simulink model "sampleModel254"  (R2021b)
settings: Solver=VariableStepAuto  StartTime=0.0  StopTime=10.0  RelTol=1e-3
undefined symbols (not defined in the file or in its folder): Newton, Raphson
libraries: simulink x14, slpidlib x3
settings Model: Creator=user  LastModifiedBy=user

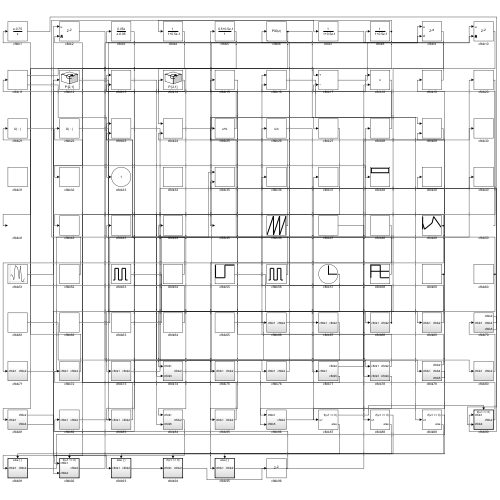
[thumbnail: Simulink's stored preview of the top-level diagram]
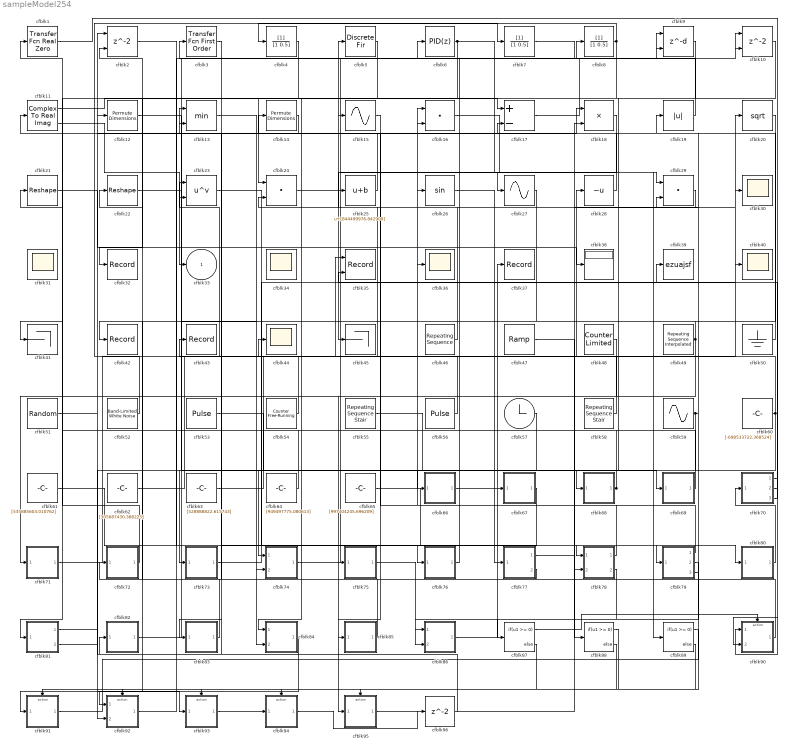
== system sampleModel254 ==
  cfblk1 : simulink/Discrete/Transfer Fcn Real Zero  ZeroZ=0.75  ICPrevInput=0.0  DoSatur=off
      settings: SourceProductBaseCode=SL
  cfblk10 : Delay  ShowEnablePort=on  SampleTime=1
      settings: InputPortMap=u0,e6
  cfblk11 : ComplexToRealImag
  cfblk12 : PermuteDimensions
  cfblk13 : MinMax  Inputs=2
  cfblk14 : PermuteDimensions
  cfblk15 : Sin  TimeSource=Use external signal  SampleTime=0
  cfblk16 : DotProduct  InputSameDT=on  OutDataTypeStr=Inherit: Inherit via internal rule
  cfblk17 : Sum  Inputs=+-
  cfblk18 : Product  Inputs=**
  cfblk19 : Abs
  cfblk2 : Delay  ShowEnablePort=on  SampleTime=1
      settings: InputPortMap=u0,e6
  cfblk20 : Sqrt  SaturateOnIntegerOverflow=on
  cfblk21 : Reshape
  cfblk22 : Reshape
  cfblk23 : Math  Operator=pow  SaturateOnIntegerOverflow=on
  cfblk24 : DotProduct  InputSameDT=on  OutDataTypeStr=Inherit: Inherit via internal rule
  cfblk25 : Bias  Bias=[844499976.842909]
  cfblk26 : Trigonometry
  cfblk27 : Sin  TimeSource=Use external signal  SampleTime=0
  cfblk28 : UnaryMinus
  cfblk29 : DotProduct  InputSameDT=on  OutDataTypeStr=Inherit: Inherit via internal rule
  cfblk3 : simulink/Discrete/Transfer Fcn First Order  PoleZ=0.95  ICPrevOutput=0.0  DoSatur=off
  cfblk{30..31,34,36,40,44} (6 alike) : Scope
      cfblk31 settings: Floating=on
      cfblk34 settings: Floating=on
  cfblk32 : Record  FileSettingsInternal="{\"entries\":[{\"content\":{\"excelSettings\":{\"content\":{},\"type\":\"Streamout.ExcelSettings\"}},\"type\":\"Streamout.FileSettingStorage\",\"uuid\":\"f8cac019-48e6-4489-905a-432bda5f2089\"}],\"packageUris\":[\"http://schema.mathworks.com/mf0/streamout_blocks/R2020a\"],\"version\":\"1.0\"}"  SignalsInternal="{\"entries\":[{\"content\":{\"signals\":[{\"content\":{\"blockPath\":[\"sampleModel254/cfblk32\"],\"channel\":[],\"dimensions\":[1],\"domain\":\"sampleModel254/cfblk32\",\"lineColor\":\"#64d413\",\"plots\":[1],\"port\":1,\"sid\":[\"\"],\"signalID\":10374,\"signalName\":\"cfblk6\"},\"type\":\"RecordBlkView.Signal\",\"uuid\":\"dce0b534-ecb6-4d5b-a233-2a280a14c64b\"}]},\"type\":\"RecordBlkView.InputSignals\",\"uuid\":\"4063d075-ef2d-4937-aee0-8c6ee8d3b7d8\"}],\"packageUris\":[\"http://schema.mathworks.com/mf0/streamout_blocks/R2020a\"],\"version\":\"1.0\"}"  VisualizationBindings="{\"sparklinesplugin\":{\"info\":[{\"bindingParametersList\":[],\"subplotID\":1}]}}"
  cfblk35 : Record  FileSettingsInternal="{\"entries\":[{\"content\":{\"excelSettings\":{\"content\":{},\"type\":\"Streamout.ExcelSettings\"}},\"type\":\"Streamout.FileSettingStorage\",\"uuid\":\"45c7964c-3e30-4dde-8807-5f474ab24dd7\"}],\"packageUris\":[\"http://schema.mathworks.com/mf0/streamout_blocks/R2020a\"],\"version\":\"1.0\"}"  Layout=[1 1]  SignalsInternal="{\"entries\":[{\"content\":{\"signals\":[{\"content\":{\"blockPath\":[\"sampleModel254/cfblk35\"],\"channel\":[],\"dimensions\":[1],\"domain\":\"sampleModel254/cfblk35\",\"lineColor\":\"#a2142f\",\"plots\":[1],\"port\":1,\"sid\":[\"\"],\"signalID\":10378,\"signalName\":\"cfblk71\"},\"type\":\"RecordBlkView.Signal\",\"uuid\":\"ef5cb758-7369-4c78-a78d-835c385c3eb8\"},{\"content\":{\"blockPath\":[\"sampleModel254/cfblk35\"],\"channel\":[],\"dimensions\":[1],\"domain\":\"sampleModel254/cfblk35\",\"lineColor\":\"#139fff\",\"plots\":[1],\"port\":2,\"sid\":[\"\"],\"signalID\":10382,\"signalName\":\"cfblk70:3\"},\"type\":\"RecordBlkView.Signal\",\"uuid\":\"7c8c1d86-132f-4531-ad7d-4a8a75f6ae5b\"}]},\"type\":\"RecordBlkView.InputSignals\",\"uuid\":\"62f64e2d-ebf5-4119-9c8a-3f565d651dbb\"}],\"packageUris\":[\"http://schema.mathworks.com/mf0/streamout_blocks/R2020a\"],\"version\":\"1.0\"}"  VisualizationBindings="{\"xyplotplugin\":{\"info\":[{\"series\":[{\"bindingParametersList\":[{\"parameter\":\"X-Axis\",\"signalID\":10378,\"signalName\":\"cfblk71\"},{\"parameter\":\"Y-Axis\",\"signalID\":10382,\"signalName\":\"cfblk70:3\"}],\"seriesID\":26922}],\"subplotID\":1}]}}"  CompatibilityTag=XY
  cfblk37 : Record  FileSettingsInternal="{\"entries\":[{\"content\":{\"excelSettings\":{\"content\":{},\"type\":\"Streamout.ExcelSettings\"}},\"type\":\"Streamout.FileSettingStorage\",\"uuid\":\"cea6e5c2-86dc-4383-be1d-b91c9e701202\"}],\"packageUris\":[\"http://schema.mathworks.com/mf0/streamout_blocks/R2020a\"],\"version\":\"1.0\"}"  SignalsInternal="{\"entries\":[{\"content\":{\"signals\":[{\"content\":{\"blockPath\":[\"sampleModel254/cfblk37\"],\"channel\":[],\"dimensions\":[1],\"domain\":\"sampleModel254/cfblk37\",\"lineColor\":\"#d95319\",\"plots\":[1],\"port\":1,\"sid\":[\"\"],\"signalID\":10394,\"signalName\":\"cfblk66\"},\"type\":\"RecordBlkView.Signal\",\"uuid\":\"769467fa-09e5-418b-a735-847f3fde8334\"}]},\"type\":\"RecordBlkView.InputSignals\",\"uuid\":\"660e46a3-809b-43d8-8dce-437cd846730a\"}],\"packageUris\":[\"http://schema.mathworks.com/mf0/streamout_blocks/R2020a\"],\"version\":\"1.0\"}"  VisualizationBindings="{\"sparklinesplugin\":{\"info\":[{\"bindingParametersList\":[],\"subplotID\":1}]}}"
  cfblk38 : Display
  cfblk39 : ToWorkspace  VariableName=ezuajsf  SaveFormat=Timeseries  SampleTime=-1
  cfblk4 : DiscreteFilter  SampleTime=1
  cfblk41 : Terminator
  cfblk42 : Record  FileSettingsInternal="{\"entries\":[{\"content\":{\"excelSettings\":{\"content\":{},\"type\":\"Streamout.ExcelSettings\"}},\"type\":\"Streamout.FileSettingStorage\",\"uuid\":\"c36e397d-8249-40e7-b36d-c436f8041f2b\"}],\"packageUris\":[\"http://schema.mathworks.com/mf0/streamout_blocks/R2020a\"],\"version\":\"1.0\"}"  SignalsInternal="{\"entries\":[{\"content\":{\"signals\":[{\"content\":{\"blockPath\":[\"sampleModel254/cfblk42\"],\"channel\":[],\"dimensions\":[1],\"domain\":\"sampleModel254/cfblk42\",\"lineColor\":\"#22b573\",\"plots\":[1],\"port\":1,\"sid\":[\"\"],\"signalID\":10386,\"signalName\":\"cfblk49\"},\"type\":\"RecordBlkView.Signal\",\"uuid\":\"95bb58e3-29ab-4543-933f-3fe3cf8075e7\"}]},\"type\":\"RecordBlkView.InputSignals\",\"uuid\":\"3d27722b-4af2-4bd2-8e99-f87c6225f507\"}],\"packageUris\":[\"http://schema.mathworks.com/mf0/streamout_blocks/R2020a\"],\"version\":\"1.0\"}"  VisualizationBindings="{\"sparklinesplugin\":{\"info\":[{\"bindingParametersList\":[],\"subplotID\":1}]}}"
  cfblk43 : Record  FileSettingsInternal="{\"entries\":[{\"content\":{\"excelSettings\":{\"content\":{},\"type\":\"Streamout.ExcelSettings\"}},\"type\":\"Streamout.FileSettingStorage\",\"uuid\":\"d18e721d-55df-43b9-9b5f-e2e7fb6a57d4\"}],\"packageUris\":[\"http://schema.mathworks.com/mf0/streamout_blocks/R2020a\"],\"version\":\"1.0\"}"  SignalsInternal="{\"entries\":[{\"content\":{\"signals\":[{\"content\":{\"blockPath\":[\"sampleModel254/cfblk43\"],\"channel\":[],\"dimensions\":[1,1],\"domain\":\"sampleModel254/cfblk43\",\"lineColor\":\"#0072bd\",\"plots\":[1],\"port\":1,\"sid\":[\"\"],\"signalID\":10390,\"signalName\":\"cfblk90\"},\"type\":\"RecordBlkView.Signal\",\"uuid\":\"5a0785be-ac31-40ab-801e-d0ec680084d0\"}]},\"type\":\"RecordBlkView.InputSignals\",\"uuid\":\"405e9301-8fb1-412e-9e94-656a63dfe870\"}],\"packageUris\":[\"http://schema.mathworks.com/mf0/streamout_blocks/R2020a\"],\"version\":\"1.0\"}"  VisualizationBindings="{\"sparklinesplugin\":{\"info\":[{\"bindingParametersList\":[],\"subplotID\":1}]}}"
  cfblk45 : Terminator
  cfblk46 : simulink/Sources/Repeating Sequence  rep_seq_t=[0 2]  rep_seq_y=[-139154258.998502, 203170849.234022]
  cfblk47 : simulink/Sources/Ramp  slope=[-2828.805781]  start=[47.728047]  InitialOutput=[-572084.834406]
  cfblk48 : simulink/Sources/Counter Limited  uplimit=[923.000000]  tsamp=-1
  cfblk49 : simulink/Sources/Repeating Sequence Interpolated  OutValues=[534969877.028503, 207347535.220771, 565089193.640656, 960177596.620139, 325028522.686949]  TimeValues=[0 0.1 0.5 0.6 1].'  LookUpMeth=Use Input Above  tsamp=0.01  OutMin=[]  OutMax=[]  OutDataTypeStr=double  OutputDataTypeScalingMode=double  OutDataType=fixdt(0,8)  OutScaling=2^-10
  cfblk5 : DiscreteFir  SampleTime=1
  cfblk50 : Ground
  cfblk51 : RandomNumber  Mean=[-71879.908599]  Variance=[65031.092299]  Seed=[190273375.000000]  SampleTime=0.1
  cfblk52 : simulink/Sources/Band-Limited White Noise  Cov=[5298985732.957167]  Ts=0.1  seed=[2012635367.000000]
  cfblk53 : DiscretePulseGenerator  PulseType=Time based  Amplitude=[128987479.442935]  Period=[95035691.423141]  PulseWidth=5  PhaseDelay=[6.000000]
  cfblk54 : simulink/Sources/Counter Free-Running  NumBits=[55.000000]  tsamp=-1
  cfblk55 : simulink/Sources/Repeating Sequence Stair  OutValues=[162166375.271766, 424616058.616663]  tsamp=-1  OutMin=[]  OutMax=[]  OutDataTypeStr=double  OutputDataTypeScalingMode=double  OutDataType=fixdt(0,8)  ConRadixGroup=Best Precision: Vector-wise  OutScaling=2^-12
  cfblk56 : DiscretePulseGenerator  PulseType=Time based  Amplitude=[530617936.673465]  Period=[21583410.222878]  PulseWidth=5  PhaseDelay=[1.000000]
  cfblk57 : Clock
  cfblk58 : simulink/Sources/Repeating Sequence Stair  OutValues=[403041999.345838, -421039062.642229]  tsamp=-1  OutMin=[]  OutMax=[]  OutDataTypeStr=double  OutputDataTypeScalingMode=double  OutDataType=fixdt(0,8)  ConRadixGroup=Best Precision: Vector-wise  OutScaling=2^-12
  cfblk59 : Sin  Amplitude=[160730542.928432]  Bias=[-895763659.447249]  SampleTime=0
  cfblk6 : slpidlib/PID Controller  Controller=PID  Form=Parallel  TimeDomain=Discrete-time  UseExternalTs=off  SampleTime=1  IntegratorMethod=Forward Euler  FilterMethod=Forward Euler  ControllerParametersSource=internal  P=1  I=1  D=0  UseFilter=on  N=100  TunerSelectOption=Transfer Function Based (PID Tuner App)  InitialConditionSource=internal  InitialConditionForIntegrator=0  InitialConditionForFilter=0  DifferentiatorICPrevScaledInput=0  ExternalReset=none  TrackingMode=off  Kt=1  LimitOutput=off  SatLimitsSource=internal  UpperSaturationLimit=inf  LowerSaturationLimit=-inf  LinearizeAsGain=off  AntiWindupMode=none  Kb=1  POutMin=[]  POutMax=[]  IOutMin=[]  IOutMax=[]  DOutMin=[]  DOutMax=[]  NOutMin=[]  NOutMax=[]  SumOutMin=[]  SumOutMax=[]  SaturationOutMin=[]  SaturationOutMax=[]  PParamMin=[]  PParamMax=[]  IParamMin=[]  IParamMax=[]  DParamMin=[]  DParamMax=[]  NParamMin=[]  NParamMax=[]  KbParamMin=[]  KbParamMax=[]  KtParamMin=[]  KtParamMax=[]  KbOutMin=[]  KbOutMax=[]  KtOutMin=[]  KtOutMax=[]  IntegratorOutMin=[]  IntegratorOutMax=[]  FilterOutMin=[]  FilterOutMax=[]  SumI1OutMin=[]  SumI1OutMax=[]  SumI2OutMin=[]  SumI2OutMax=[]  SumI3OutMin=[]  SumI3OutMax=[]  SumI4OutMin=[]  SumI4OutMax=[]  SumDOutMin=[]  SumDOutMax=[]  DifferentiatorOutMin=[]  DifferentiatorOutMax=[]  FilterDiffOutCoefMin=[]  FilterDiffOutCoefMax=[]  ReciprocalOutMin=[]  ReciprocalOutMax=[]  SumDenOutMin=[]  SumDenOutMax=[]  SumNumOutMin=[]  SumNumOutMax=[]  DivideOutMin=[]  DivideOutMax=[]  UdiffTsProdOutMin=[]  UdiffTsProdOutMax=[]  NTsProdOutMin=[]  NTsProdOutMax=[]  UintegralTsProdOutMin=[]  UintegralTsProdOutMax=[]  UngainTsProdOutMin=[]  UngainTsProdOutMax=[]  IntegratorContinuousStateAttributes=''  IntegratorStateMustResolveToSignalObject=off  IntegratorRTWStateStorageClass=Auto  FilterContinuousStateAttributes=''  FilterStateMustResolveToSignalObject=off  FilterRTWStateStorageClass=Auto  ParallelPVariant=InternalParameters  IdealPVariant=Disabled  IVariant=InternalParameters  DVariant=InternalParameters  IntegratorVariant=Discrete  SatVariant=Disabled  AWVariant=Passthrough  PCopyVariant=Disabled  TRVariant=Disabled  FdbkBlocksVariant=Forward  IdealPFdbkVariant=Disabled  SatFdbkVariant=Disabled  DerivativeFilterVariant=ForwardEulerFilter  NVariant=InternalParameters  NCopyVariant=Disabled  FilterICVariant=InternalICsFilter  IntegratorICVariant=InternalICs  ExternalResetVariant=Disabled  TRSumVariant=Passthrough  SumFdbkVariant=Disabled  SumVariant=Sum_PID  TsampFilterVariant=InternalTs  TsampNgainVariant=Passthrough  TsampIntegralVariant=Passthrough  ExternalSaturationOutDataTypeStr=Inherit: Same as second input
  cfblk60 : Constant  Value=[-698533722.368524]  SampleTime=1
  cfblk61 : Constant  Value=[535885603.010762]  SampleTime=1
  cfblk62 : Constant  Value=[305687430.388225]  SampleTime=1
  cfblk63 : Constant  Value=[528888822.615743]  SampleTime=1
  cfblk64 : Constant  Value=[949497775.080613]  SampleTime=1
  cfblk65 : Constant  Value=[997404245.696209]  SampleTime=1
  cfblk66 : Subsystem
  cfblk67 : Subsystem
  cfblk68 : Subsystem
  cfblk69 : Subsystem
  cfblk7 : DiscreteFilter  SampleTime=1
  cfblk70 : Subsystem
  cfblk71 : Subsystem
  cfblk72 : Subsystem
  cfblk73 : Subsystem
  cfblk74 : Subsystem
  cfblk75 : Subsystem
  cfblk76 : Subsystem
  cfblk77 : Subsystem
  cfblk78 : Subsystem
  cfblk79 : Subsystem
  cfblk8 : DiscreteFilter  SampleTime=1
  cfblk80 : Subsystem
  cfblk81 : Subsystem
  cfblk82 : Subsystem
  cfblk83 : Subsystem
  cfblk84 : Subsystem
  cfblk85 : Subsystem
  cfblk86 : Subsystem
  cfblk87 : If  IfExpression=u1 >= 0  SampleTime=1
  cfblk88 : If  IfExpression=u1 >= 0  SampleTime=1
  cfblk89 : If  IfExpression=u1 >= 0  SampleTime=1
  cfblk9 : Delay  DelayLengthSource=Input port  SampleTime=1
      settings: InputPortMap=u0,p1
  cfblk90 : Subsystem  TreatAsAtomicUnit=on
  cfblk91 : Subsystem  TreatAsAtomicUnit=on
  cfblk92 : Subsystem  TreatAsAtomicUnit=on
  cfblk93 : Subsystem  TreatAsAtomicUnit=on
  cfblk94 : Subsystem  TreatAsAtomicUnit=on
  cfblk95 : Subsystem  TreatAsAtomicUnit=on
  cfblk96 : Delay  SampleTime=1
  cfblk33 : Outport
  wires:
  cfblk82/1(cfblk2) -> cfblk10/1
  cfblk67/1(cfblk2) -> cfblk82/1(cfblk1)
  cfblk93/1(cfblk2) -> cfblk94/1(cfblk1)
  cfblk49/1 -> cfblk42/1, cfblk71/1(cfblk1)
  cfblk12/1 -> cfblk69/1(cfblk1)
  cfblk57/1 -> cfblk73/1(cfblk1)
  cfblk24/1 -> cfblk27/1
  cfblk50/1 -> cfblk19/1
  cfblk74/1(cfblk2) -> cfblk8/1
  cfblk62/1 -> cfblk28/1
  cfblk91/1(cfblk2) -> cfblk39/1
  cfblk66/1(cfblk2) -> cfblk37/1
  cfblk90/1(cfblk2) -> cfblk43/1
  cfblk9/1 -> cfblk68/1(cfblk1)
  cfblk3/1 -> cfblk83/1(cfblk1)
  cfblk83/1(cfblk2) -> cfblk22/1
  cfblk68/1(cfblk2) -> cfblk16/1, cfblk6/1
  cfblk18/1 -> cfblk45/1
  cfblk19/1 -> cfblk3/1
  cfblk63/1 -> cfblk20/1
  cfblk52/1 -> cfblk7/1
  cfblk61/1 -> cfblk76/1(cfblk1)
  cfblk64/1 -> cfblk13/1
  cfblk10/1 -> cfblk24/1
  cfblk79/1(cfblk2) -> cfblk26/1
  cfblk48/1 -> cfblk95/1(cfblk1)
  cfblk46/1 -> cfblk5/1
  cfblk25/1 -> cfblk11/1
  cfblk1/1 -> cfblk90/1(cfblk1)
  cfblk73/1(cfblk2) -> cfblk40/1
  cfblk81/1(cfblk2) -> cfblk93/1(cfblk1)
  cfblk23/1 -> cfblk80/1(cfblk1)
  cfblk92/1(cfblk2) -> cfblk10/2
  cfblk54/1 -> cfblk44/1
  cfblk60/1 -> cfblk74/1(cfblk1), cfblk23/2
  cfblk11/1 -> cfblk17/1
  cfblk71/1(cfblk2) -> cfblk35/1
  cfblk17/1 -> cfblk9/1
  cfblk28/1 -> cfblk14/1
  cfblk65/1 -> cfblk78/1(cfblk1)
  cfblk13/1 -> cfblk75/1(cfblk1)
  cfblk69/1(cfblk2) -> cfblk1/1
  cfblk21/1 -> cfblk38/1
  cfblk47/1 -> cfblk78/2(cfblk3)
  cfblk58/1 -> cfblk25/1
  cfblk70/1(cfblk2) -> cfblk90/2(cfblk4)
  cfblk2/1 -> cfblk79/1(cfblk1)
  cfblk14/1 -> cfblk13/2
  cfblk51/1 -> cfblk12/1
  cfblk81/2(cfblk4) -> cfblk18/1
  cfblk16/1 -> cfblk89/1
  cfblk4/1 -> cfblk41/1
  cfblk86/1(cfblk2) -> cfblk67/1(cfblk1)
  cfblk80/1(cfblk2) -> cfblk70/1(cfblk1)
  cfblk79/2(cfblk4) -> cfblk87/1
  cfblk76/1(cfblk2) -> cfblk16/2
  cfblk5/1 -> cfblk84/1(cfblk1)
  cfblk6/1 -> cfblk32/1, cfblk29/1
  cfblk70/2(cfblk4) -> cfblk36/1
  cfblk8/1 -> cfblk81/1(cfblk1), cfblk4/1
  cfblk27/1 -> cfblk74/2(cfblk3)
  cfblk84/1(cfblk2) -> cfblk91/1(cfblk1)
  cfblk85/1(cfblk2) -> cfblk2/2
  cfblk20/1 -> cfblk92/1(cfblk1)
  cfblk75/1(cfblk2) -> cfblk86/1(cfblk1)
  cfblk22/1 -> cfblk84/2(cfblk5)
  cfblk79/3(cfblk5) -> cfblk17/2
  cfblk26/1 -> cfblk77/1(cfblk1)
  cfblk70/3(cfblk5) -> cfblk35/2
  cfblk53/1 -> cfblk66/1(cfblk1)
  cfblk15/1 -> cfblk85/1(cfblk1)
  cfblk95/1(cfblk2) -> cfblk18/2
  cfblk11/2 -> cfblk33/1
  cfblk72/1(cfblk2) -> cfblk21/1
  cfblk29/1 -> cfblk24/2
  cfblk55/1 -> cfblk88/1
  cfblk56/1 -> cfblk23/1
  cfblk78/1(cfblk2) -> cfblk15/1
  cfblk77/1(cfblk2) -> cfblk30/1
  cfblk7/1 -> cfblk9/2
  cfblk59/1 -> cfblk92/2(cfblk4), cfblk29/2
  cfblk78/2(cfblk4) -> cfblk86/2(cfblk5)
  cfblk77/2(cfblk5) -> cfblk72/1(cfblk1)
  cfblk87/1 -> cfblk90/Action
  cfblk87/2 -> cfblk91/Action
  cfblk88/1 -> cfblk92/Action
  cfblk88/2 -> cfblk93/Action
  cfblk89/1 -> cfblk94/Action
  cfblk89/2 -> cfblk95/Action
  cfblk94/1(cfblk2) -> cfblk96/1
  cfblk96/1 -> cfblk2/1

== system sampleModel254/cfblk66 ==
  cfblk1 : Inport
  cfblk3 : simulink/Discrete/Transfer Fcn Real Zero  ZeroZ=0.75  ICPrevInput=0.0  DoSatur=off
      settings: SourceProductBaseCode=SL
  cfblk2 : Outport
  wires:
  cfblk3/1 -> cfblk2/1
  cfblk1/1 -> cfblk3/1

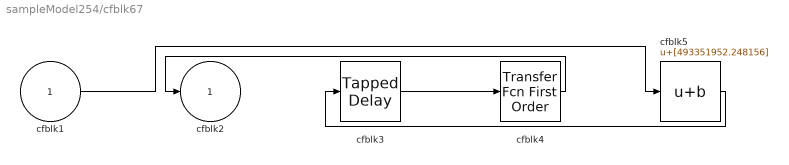
== system sampleModel254/cfblk67 ==
  cfblk1 : Inport
  cfblk3 : simulink/Discrete/Tapped Delay  vinit=0.0  samptime=-1  NumDelays=1  DelayOrder=Oldest  includeCurrent=off
  cfblk4 : simulink/Discrete/Transfer Fcn First Order  PoleZ=0.95  ICPrevOutput=0.0  DoSatur=off
  cfblk5 : Bias  Bias=[493351952.248156]
  cfblk2 : Outport
  wires:
  cfblk4/1 -> cfblk2/1
  cfblk5/1 -> cfblk3/1
  cfblk1/1 -> cfblk5/1
  cfblk3/1 -> cfblk4/1

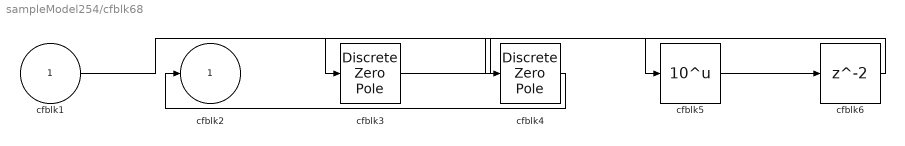
== system sampleModel254/cfblk68 ==
  cfblk1 : Inport
  cfblk3 : DiscreteZeroPole  Poles=[0 0.5]  Gain=1
  cfblk4 : DiscreteZeroPole  Poles=[0 0.5]  Gain=1
  cfblk5 : Math  Operator=10^u  SaturateOnIntegerOverflow=on
  cfblk6 : Delay  SampleTime=1
  cfblk2 : Outport
  wires:
  cfblk3/1 -> cfblk5/1
  cfblk4/1 -> cfblk2/1
  cfblk1/1 -> cfblk4/1
  cfblk5/1 -> cfblk6/1
  cfblk6/1 -> cfblk3/1

== system sampleModel254/cfblk69 ==
  cfblk1 : Inport
  cfblk3 : ComplexToRealImag
  cfblk2 : Outport
  wires:
  cfblk1/1 -> cfblk3/1
  cfblk3/1 -> cfblk2/1

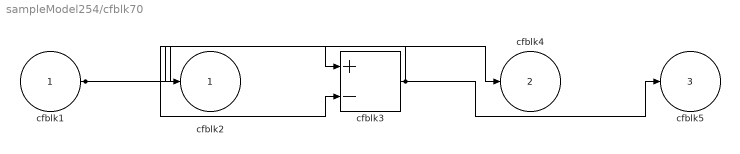
== system sampleModel254/cfblk70 ==
  cfblk1 : Inport
  cfblk3 : Sum  Inputs=+-
  cfblk2 : Outport
  cfblk4 : Outport  Port=2
  cfblk5 : Outport  Port=3
  wires:
  cfblk1/1 -> cfblk4/1, cfblk3/1, cfblk3/2
  cfblk3/1 -> cfblk5/1, cfblk2/1

== system sampleModel254/cfblk71 ==
  cfblk1 : Inport
  cfblk3 : UnaryMinus
  cfblk2 : Outport
  wires:
  cfblk3/1 -> cfblk2/1
  cfblk1/1 -> cfblk3/1

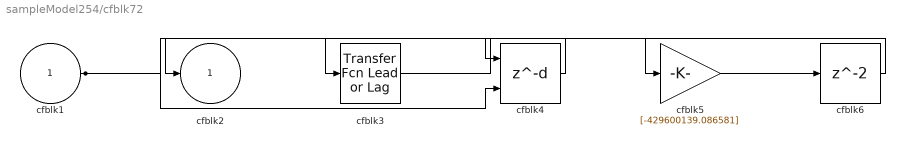
== system sampleModel254/cfblk72 ==
  cfblk1 : Inport
  cfblk3 : simulink/Discrete/Transfer Fcn Lead or Lag  PoleZ=0.95  ZeroZ=0.75  ICPrevOutput=0.0  ICPrevInput=0.0  DoSatur=off
      settings: SourceProductBaseCode=SL
  cfblk4 : Delay  DelayLengthSource=Input port  SampleTime=1
      settings: InputPortMap=u0,p1
  cfblk5 : Gain  Gain=[-429600139.086581]
  cfblk6 : Delay  SampleTime=1
  cfblk2 : Outport
  wires:
  cfblk3/1 -> cfblk5/1
  cfblk4/1 -> cfblk2/1
  cfblk1/1 -> cfblk4/1, cfblk4/2
  cfblk5/1 -> cfblk6/1
  cfblk6/1 -> cfblk3/1

== system sampleModel254/cfblk73 ==
  cfblk1 : Inport
  cfblk3 : Abs
  cfblk2 : Outport
  wires:
  cfblk1/1 -> cfblk2/1, cfblk3/1

== system sampleModel254/cfblk74 ==
  cfblk1 : Inport
  cfblk3 : Inport  Port=2
  cfblk2 : Outport
  wires:
  cfblk1/1 -> cfblk2/1

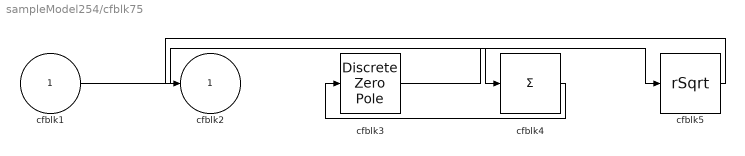
== system sampleModel254/cfblk75 ==
  cfblk1 : Inport
  cfblk3 : DiscreteZeroPole  Poles=[0 0.5]  Gain=1
  cfblk4 : Sum  Inputs=+
  cfblk5 : Sqrt  Operator=rSqrt  AlgorithmType=Newton-Raphson  SaturateOnIntegerOverflow=on
  cfblk2 : Outport
  wires:
  cfblk1/1 -> cfblk4/1
  cfblk4/1 -> cfblk3/1
  cfblk3/1 -> cfblk5/1
  cfblk5/1 -> cfblk2/1

== system sampleModel254/cfblk76 ==
  cfblk1 : Inport
  cfblk3 : Delay  DelayLengthSource=Input port  SampleTime=1
      settings: InputPortMap=u0,p1
  cfblk4 : Constant  Value=[439101248.197444]  SampleTime=1
  cfblk2 : Outport
  wires:
  cfblk1/1 -> cfblk3/1
  cfblk3/1 -> cfblk2/1
  cfblk4/1 -> cfblk3/2

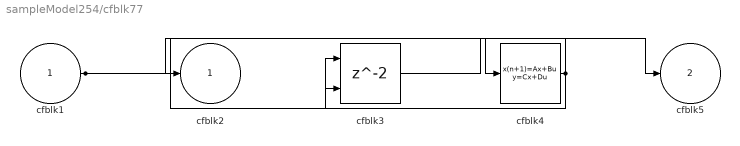
== system sampleModel254/cfblk77 ==
  cfblk1 : Inport
  cfblk3 : Delay  ShowEnablePort=on  SampleTime=1
      settings: InputPortMap=u0,e6
  cfblk4 : DiscreteStateSpace
  cfblk2 : Outport
  cfblk5 : Outport  Port=2
  wires:
  cfblk1/1 -> cfblk4/1, cfblk3/2
  cfblk4/1 -> cfblk3/1, cfblk2/1
  cfblk3/1 -> cfblk5/1

== system sampleModel254/cfblk78 ==
  cfblk1 : Inport
  cfblk3 : Inport  Port=2
  cfblk2 : Outport
  cfblk4 : Outport  Port=2
  wires:
  cfblk1/1 -> cfblk4/1
  cfblk3/1 -> cfblk2/1

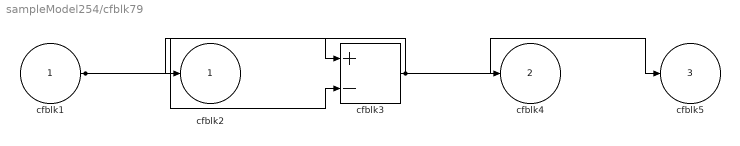
== system sampleModel254/cfblk79 ==
  cfblk1 : Inport
  cfblk3 : Sum  Inputs=+-
  cfblk2 : Outport
  cfblk4 : Outport  Port=2
  cfblk5 : Outport  Port=3
  wires:
  cfblk1/1 -> cfblk3/1, cfblk3/2
  cfblk3/1 -> cfblk5/1, cfblk4/1, cfblk2/1

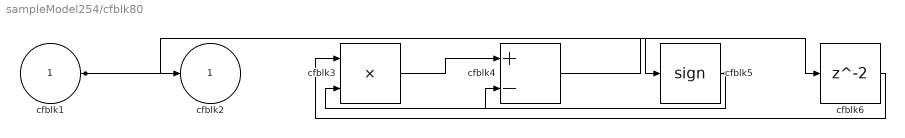
== system sampleModel254/cfblk80 ==
  cfblk1 : Inport
  cfblk3 : Product
  cfblk4 : Sum  Inputs=+-
  cfblk5 : Signum
  cfblk6 : Delay  SampleTime=1
  cfblk2 : Outport
  wires:
  cfblk1/1 -> cfblk2/1, cfblk5/1
  cfblk5/1 -> cfblk3/2, cfblk4/2
  cfblk3/1 -> cfblk4/1
  cfblk4/1 -> cfblk6/1
  cfblk6/1 -> cfblk3/1

== system sampleModel254/cfblk81 ==
  cfblk1 : Inport
  cfblk3 : Constant  Value=[316923812.168130]  SampleTime=1
  cfblk2 : Outport
  cfblk4 : Outport  Port=2
  wires:
  cfblk3/1 -> cfblk2/1
  cfblk1/1 -> cfblk4/1

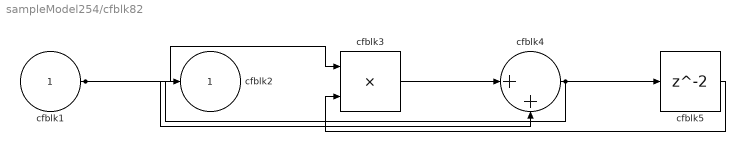
== system sampleModel254/cfblk82 ==
  cfblk1 : Inport
  cfblk3 : Product
  cfblk4 : Sum  Inputs=|++
  cfblk5 : Delay  SampleTime=1
  cfblk2 : Outport
  wires:
  cfblk1/1 -> cfblk3/1, cfblk4/2
  cfblk3/1 -> cfblk4/1
  cfblk4/1 -> cfblk2/1, cfblk5/1
  cfblk5/1 -> cfblk3/2

== system sampleModel254/cfblk83 ==
  cfblk1 : Inport
  cfblk3 : PermuteDimensions
  cfblk4 : Signum
  cfblk2 : Outport
  wires:
  cfblk1/1 -> cfblk3/1
  cfblk3/1 -> cfblk4/1
  cfblk4/1 -> cfblk2/1

== system sampleModel254/cfblk84 ==
  cfblk1 : Inport
  cfblk5 : Inport  Port=2
  cfblk3 : slpidlib/PID Controller (2DOF)  Controller=PID  Form=Parallel  TimeDomain=Discrete-time  UseExternalTs=off  SampleTime=1  IntegratorMethod=Forward Euler  FilterMethod=Forward Euler  ControllerParametersSource=internal  P=1  I=1  D=0  UseFilter=on  N=100  b=1  c=1  TunerSelectOption=Transfer Function Based (PID Tuner App)  InitialConditionSource=internal  InitialConditionForIntegrator=0  InitialConditionForFilter=0  DifferentiatorICPrevScaledInput=0  ExternalReset=none  TrackingMode=off  Kt=1  LimitOutput=off  SatLimitsSource=internal  UpperSaturationLimit=inf  LowerSaturationLimit=-inf  LinearizeAsGain=off  AntiWindupMode=none  Kb=1  POutMin=[]  POutMax=[]  IOutMin=[]  IOutMax=[]  DOutMin=[]  DOutMax=[]  NOutMin=[]  NOutMax=[]  bOutMin=[]  bOutMax=[]  cOutMin=[]  cOutMax=[]  SumOutMin=[]  SumOutMax=[]  SaturationOutMin=[]  SaturationOutMax=[]  PParamMin=[]  PParamMax=[]  IParamMin=[]  IParamMax=[]  DParamMin=[]  DParamMax=[]  NParamMin=[]  NParamMax=[]  bParamMin=[]  bParamMax=[]  cParamMin=[]  cParamMax=[]  KbParamMin=[]  KbParamMax=[]  KtParamMin=[]  KtParamMax=[]  KbOutMin=[]  KbOutMax=[]  KtOutMin=[]  KtOutMax=[]  IntegratorOutMin=[]  IntegratorOutMax=[]  FilterOutMin=[]  FilterOutMax=[]  SumI1OutMin=[]  SumI1OutMax=[]  SumI2OutMin=[]  SumI2OutMax=[]  SumI3OutMin=[]  SumI3OutMax=[]  SumI4OutMin=[]  SumI4OutMax=[]  SumDOutMin=[]  SumDOutMax=[]  Sum1OutMin=[]  Sum1OutMax=[]  Sum2OutMin=[]  Sum2OutMax=[]  Sum3OutMin=[]  Sum3OutMax=[]  DifferentiatorOutMin=[]  DifferentiatorOutMax=[]  FilterDiffOutCoefMin=[]  FilterDiffOutCoefMax=[]  ReciprocalOutMin=[]  ReciprocalOutMax=[]  SumDenOutMin=[]  SumDenOutMax=[]  SumNumOutMin=[]  SumNumOutMax=[]  DivideOutMin=[]  DivideOutMax=[]  UdiffTsProdOutMin=[]  UdiffTsProdOutMax=[]  NTsProdOutMin=[]  NTsProdOutMax=[]  UintegralTsProdOutMin=[]  UintegralTsProdOutMax=[]  UngainTsProdOutMin=[]  UngainTsProdOutMax=[]  IntegratorContinuousStateAttributes=''  IntegratorStateMustResolveToSignalObject=off  IntegratorRTWStateStorageClass=Auto  FilterContinuousStateAttributes=''  FilterStateMustResolveToSignalObject=off  FilterRTWStateStorageClass=Auto  ParallelPVariant=InternalParameters  IdealPVariant=Disabled  IVariant=InternalParameters  DVariant=InternalParameters  bVariant=InternalParameters  cVariant=InternalParameters  IntegratorVariant=Discrete  SatVariant=Disabled  AWVariant=Passthrough  PCopyVariant=Disabled  TRVariant=Disabled  FdbkBlocksVariant=Forward  IdealPFdbkVariant=Disabled  SatFdbkVariant=Disabled  DerivativeFilterVariant=ForwardEulerFilter  NVariant=InternalParameters  NCopyVariant=Disabled  FilterICVariant=InternalICsFilter  IntegratorICVariant=InternalICs  ExternalResetVariant=Disabled  TRSumVariant=Passthrough  SumFdbkVariant=Disabled  SumVariant=Sum_PID  TsampFilterVariant=InternalTs  TsampNgainVariant=Passthrough  TsampIntegralVariant=Passthrough  ExternalSaturationOutDataTypeStr=Inherit: Same as second input
      settings: SourceProductBaseCode=SL
  cfblk4 : Constant  Value=[-675125384.353704]  SampleTime=1
  cfblk2 : Outport
  wires:
  cfblk4/1 -> cfblk2/1
  cfblk5/1 -> cfblk3/1
  cfblk1/1 -> cfblk3/2

== system sampleModel254/cfblk85 ==
  cfblk1 : Inport
  cfblk3 : Delay  ShowEnablePort=on  SampleTime=1
      settings: InputPortMap=u0,e6
  cfblk2 : Outport
  wires:
  cfblk1/1 -> cfblk3/1, cfblk3/2
  cfblk3/1 -> cfblk2/1

== system sampleModel254/cfblk86 ==
  cfblk1 : Inport
  cfblk5 : Inport  Port=2
  cfblk3 : DiscreteFir  SampleTime=1
  cfblk4 : DiscreteTransferFcn  SampleTime=1
  cfblk2 : Outport
  wires:
  cfblk3/1 -> cfblk2/1
  cfblk5/1 -> cfblk4/1
  cfblk1/1 -> cfblk3/1

== system sampleModel254/cfblk90 ==
  cfblk1 : Inport
  cfblk4 : Inport  Port=2
  Action Port : ActionPort  ActionPortLabel=if(u1 >= 0)
  cfblk3 : Sqrt  SaturateOnIntegerOverflow=on
  cfblk2 : Outport
  wires:
  cfblk1/1 -> cfblk3/1
  cfblk3/1 -> cfblk2/1

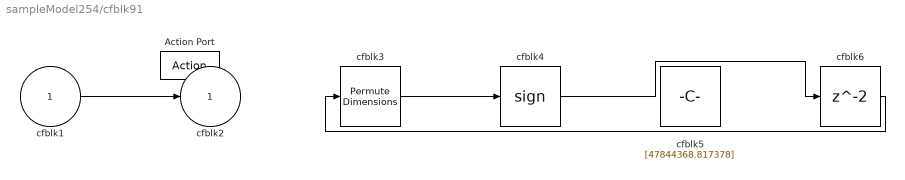
== system sampleModel254/cfblk91 ==
  cfblk1 : Inport
  Action Port : ActionPort  ActionPortLabel=else
  cfblk3 : PermuteDimensions
  cfblk4 : Signum
  cfblk5 : Constant  Value=[47844368.817378]  SampleTime=1
  cfblk6 : Delay
  cfblk2 : Outport
  wires:
  cfblk3/1 -> cfblk4/1
  cfblk1/1 -> cfblk2/1
  cfblk4/1 -> cfblk6/1
  cfblk6/1 -> cfblk3/1

== system sampleModel254/cfblk92 ==
  cfblk1 : Inport
  cfblk4 : Inport  Port=2
  Action Port : ActionPort  ActionPortLabel=if(u1 >= 0)
  cfblk3 : Sum  Inputs=|++
  cfblk2 : Outport
  wires:
  cfblk3/1 -> cfblk2/1
  cfblk1/1 -> cfblk3/1
  cfblk4/1 -> cfblk3/2

== system sampleModel254/cfblk93 ==
  cfblk1 : Inport
  Action Port : ActionPort  ActionPortLabel=else
  cfblk3 : Delay
  cfblk2 : Outport
  wires:
  cfblk1/1 -> cfblk3/1
  cfblk3/1 -> cfblk2/1

== system sampleModel254/cfblk94 ==
  cfblk1 : Inport
  Action Port : ActionPort  ActionPortLabel=if(u1 >= 0)
  cfblk3 : slpidlib/PID Controller  Controller=PID  Form=Parallel  TimeDomain=Discrete-time  UseExternalTs=off  SampleTime=-1  IntegratorMethod=Forward Euler  FilterMethod=Forward Euler  ControllerParametersSource=internal  P=1  I=1  D=0  UseFilter=on  N=100  TunerSelectOption=Transfer Function Based (PID Tuner App)  InitialConditionSource=internal  InitialConditionForIntegrator=0  InitialConditionForFilter=0  DifferentiatorICPrevScaledInput=0  ExternalReset=none  TrackingMode=off  Kt=1  LimitOutput=off  SatLimitsSource=internal  UpperSaturationLimit=inf  LowerSaturationLimit=-inf  LinearizeAsGain=off  AntiWindupMode=none  Kb=1  POutMin=[]  POutMax=[]  IOutMin=[]  IOutMax=[]  DOutMin=[]  DOutMax=[]  NOutMin=[]  NOutMax=[]  SumOutMin=[]  SumOutMax=[]  SaturationOutMin=[]  SaturationOutMax=[]  PParamMin=[]  PParamMax=[]  IParamMin=[]  IParamMax=[]  DParamMin=[]  DParamMax=[]  NParamMin=[]  NParamMax=[]  KbParamMin=[]  KbParamMax=[]  KtParamMin=[]  KtParamMax=[]  KbOutMin=[]  KbOutMax=[]  KtOutMin=[]  KtOutMax=[]  IntegratorOutMin=[]  IntegratorOutMax=[]  FilterOutMin=[]  FilterOutMax=[]  SumI1OutMin=[]  SumI1OutMax=[]  SumI2OutMin=[]  SumI2OutMax=[]  SumI3OutMin=[]  SumI3OutMax=[]  SumI4OutMin=[]  SumI4OutMax=[]  SumDOutMin=[]  SumDOutMax=[]  DifferentiatorOutMin=[]  DifferentiatorOutMax=[]  FilterDiffOutCoefMin=[]  FilterDiffOutCoefMax=[]  ReciprocalOutMin=[]  ReciprocalOutMax=[]  SumDenOutMin=[]  SumDenOutMax=[]  SumNumOutMin=[]  SumNumOutMax=[]  DivideOutMin=[]  DivideOutMax=[]  UdiffTsProdOutMin=[]  UdiffTsProdOutMax=[]  NTsProdOutMin=[]  NTsProdOutMax=[]  UintegralTsProdOutMin=[]  UintegralTsProdOutMax=[]  UngainTsProdOutMin=[]  UngainTsProdOutMax=[]  IntegratorContinuousStateAttributes=''  IntegratorStateMustResolveToSignalObject=off  IntegratorRTWStateStorageClass=Auto  FilterContinuousStateAttributes=''  FilterStateMustResolveToSignalObject=off  FilterRTWStateStorageClass=Auto  ParallelPVariant=InternalParameters  IdealPVariant=Disabled  IVariant=InternalParameters  DVariant=InternalParameters  IntegratorVariant=Discrete  SatVariant=Disabled  AWVariant=Passthrough  PCopyVariant=Disabled  TRVariant=Disabled  FdbkBlocksVariant=Forward  IdealPFdbkVariant=Disabled  SatFdbkVariant=Disabled  DerivativeFilterVariant=ForwardEulerFilter  NVariant=InternalParameters  NCopyVariant=Disabled  FilterICVariant=InternalICsFilter  IntegratorICVariant=InternalICs  ExternalResetVariant=Disabled  TRSumVariant=Passthrough  SumFdbkVariant=Disabled  SumVariant=Sum_PID  TsampFilterVariant=InternalTs  TsampNgainVariant=Passthrough  TsampIntegralVariant=Passthrough  ExternalSaturationOutDataTypeStr=Inherit: Same as second input
  cfblk4 : Sum  Inputs=+-
  cfblk2 : Outport
  wires:
  cfblk1/1 -> cfblk3/1
  cfblk3/1 -> cfblk4/1, cfblk4/2
  cfblk4/1 -> cfblk2/1

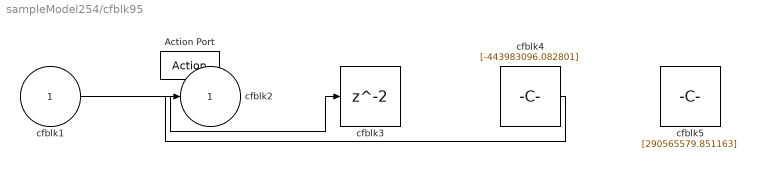
== system sampleModel254/cfblk95 ==
  cfblk1 : Inport
  Action Port : ActionPort  ActionPortLabel=else
  cfblk3 : Delay
  cfblk4 : Constant  Value=[-443983096.082801]  SampleTime=1
  cfblk5 : Constant  Value=[290565579.851163]  SampleTime=1
  cfblk2 : Outport
  wires:
  cfblk1/1 -> cfblk3/1
  cfblk4/1 -> cfblk2/1
